simulink model "ideal_ballnbeam"  (R2020b)
settings: Solver=ode15s  StartTime=0.0  StopTime=100  RelTol=1e-3
undefined symbols (not defined in the file): ball, ballnbeam, const, mech
settings Model: Creator=Utente  LastModifiedBy=Utente

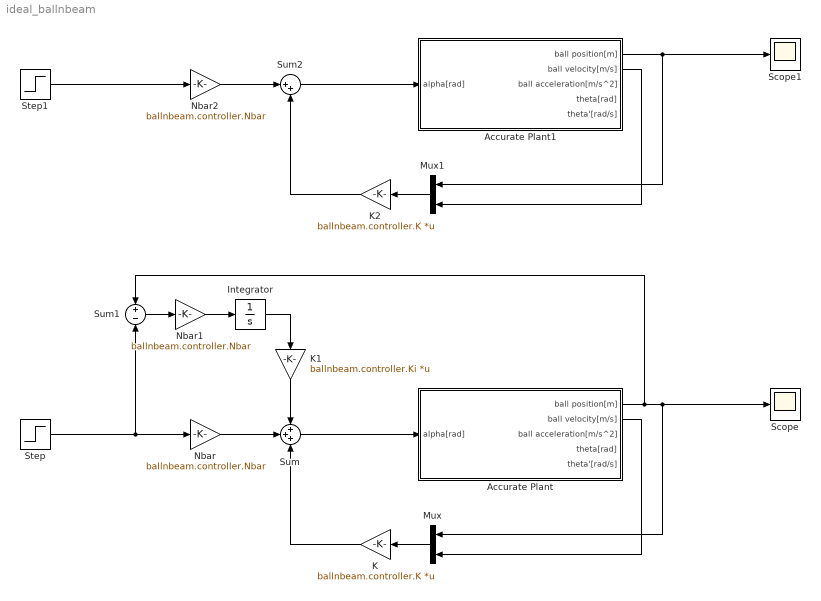
== system ideal_ballnbeam ==
  Accurate Plant : Subsystem
  Accurate Plant1 : Subsystem
  Integrator : Integrator
  K : Gain  Gain=ballnbeam.controller.K  Multiplication=Matrix(K*u)
  K1 : Gain  Gain=ballnbeam.controller.Ki  Multiplication=Matrix(K*u)
  K2 : Gain  Gain=ballnbeam.controller.K  Multiplication=Matrix(K*u)
  Mux : Mux  Inputs=2
  Mux1 : Mux  Inputs=2
  Nbar : Gain  Gain=ballnbeam.controller.Nbar
  Nbar1 : Gain  Gain=ballnbeam.controller.Nbar
  Nbar2 : Gain  Gain=ballnbeam.controller.Nbar
  Scope : Scope
  Scope1 : Scope
  Step : Step  Time=0  After=0.25  SampleTime=0
  Step1 : Step  Time=0  After=0.25  SampleTime=0
  Sum : Sum  Inputs=+++
  Sum1 : Sum  Inputs=+|-
  Sum2 : Sum  Inputs=|++
  wires:
  Accurate Plant/1(ball position[m]) -> Mux/1, Scope/1, Sum1/1
  Sum/1 -> Accurate Plant/1(alpha[rad])
  Mux/1 -> K/1
  Accurate Plant/2(ball velocity[m/s]) -> Mux/2
  Sum1/1 -> Nbar1/1
  Integrator/1 -> K1/1
  K/1 -> Sum/3
  Step/1 -> Nbar/1, Sum1/2
  K1/1 -> Sum/1
  Nbar1/1 -> Integrator/1
  Nbar/1 -> Sum/2
  Step1/1 -> Nbar2/1
  K2/1 -> Sum2/2
  Accurate Plant1/1(ball position[m]) -> Mux1/1, Scope1/1
  Accurate Plant1/2(ball velocity[m/s]) -> Mux1/2
  Sum2/1 -> Accurate Plant1/1(alpha[rad])
  Mux1/1 -> K2/1
  Nbar2/1 -> Sum2/1

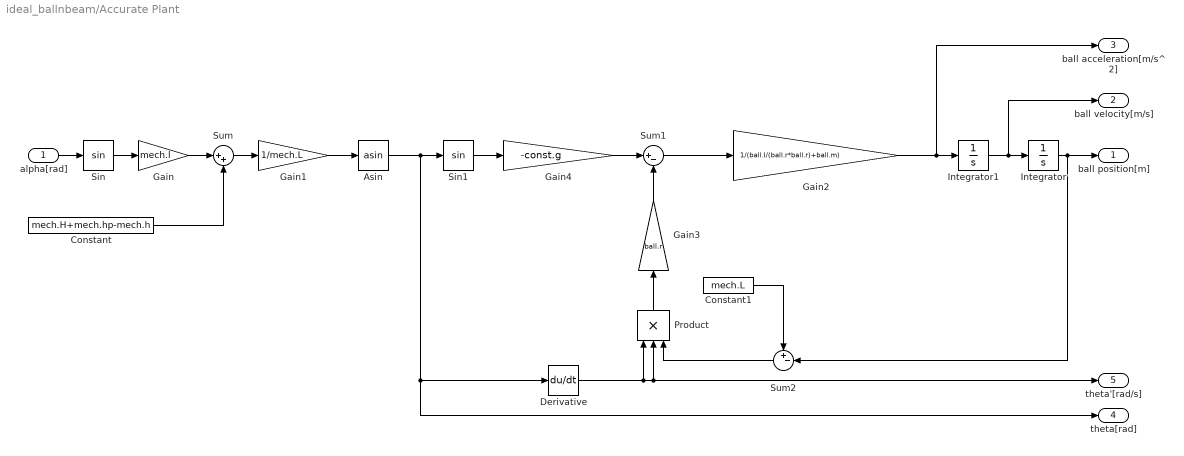
== system ideal_ballnbeam/Accurate Plant ==
  alpha[rad] : Inport
  Asin : Trigonometry  Operator=asin
  Constant : Constant  Value=mech.H+mech.hp-mech.h
  Constant1 : Constant  Value=mech.L
  Derivative : Derivative
  Gain : Gain  Gain=mech.l
  Gain1 : Gain  Gain=1/mech.L
  Gain2 : Gain  Gain=1/(ball.I/(ball.r*ball.r)+ball.m)
  Gain3 : Gain  Gain=ball.r
  Gain4 : Gain  Gain=-const.g
  Integrator : Integrator
  Integrator1 : Integrator
  Product : Product  Inputs=3
  Sin : Trigonometry
  Sin1 : Trigonometry
  Sum : Sum  Inputs=|++
  Sum1 : Sum  Inputs=|+-
  Sum2 : Sum  Inputs=+-|
  ball position[m] : Outport
  ball velocity[m/s] : Outport  Port=2
  ball acceleration[m/s^2] : Outport  Port=3
  theta[rad] : Outport  Port=4
  theta'[rad/s] : Outport  Port=5
  wires:
  Integrator/1 -> Sum2/2, ball position[m]/1
  Integrator1/1 -> ball velocity[m/s]/1, Integrator/1
  Gain2/1 -> ball acceleration[m/s^2]/1, Integrator1/1
  Gain1/1 -> Asin/1
  Gain/1 -> Sum/1
  Sum/1 -> Gain1/1
  alpha[rad]/1 -> Sin/1
  Constant/1 -> Sum/2
  Sin/1 -> Gain/1
  Asin/1 -> Derivative/1, theta[rad]/1, Sin1/1
  Derivative/1 -> Product/1, theta'[rad/s]/1, Product/2
  Product/1 -> Gain3/1
  Gain3/1 -> Sum1/2
  Sum1/1 -> Gain2/1
  Sin1/1 -> Gain4/1
  Gain4/1 -> Sum1/1
  Sum2/1 -> Product/3
  Constant1/1 -> Sum2/1

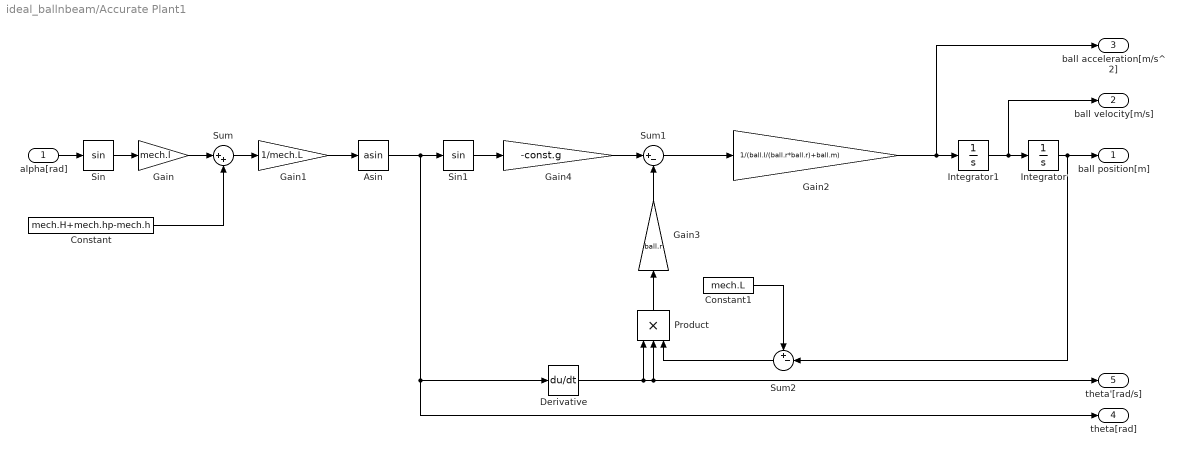
== system ideal_ballnbeam/Accurate Plant1 ==
  alpha[rad] : Inport
  Asin : Trigonometry  Operator=asin
  Constant : Constant  Value=mech.H+mech.hp-mech.h
  Constant1 : Constant  Value=mech.L
  Derivative : Derivative
  Gain : Gain  Gain=mech.l
  Gain1 : Gain  Gain=1/mech.L
  Gain2 : Gain  Gain=1/(ball.I/(ball.r*ball.r)+ball.m)
  Gain3 : Gain  Gain=ball.r
  Gain4 : Gain  Gain=-const.g
  Integrator : Integrator
  Integrator1 : Integrator
  Product : Product  Inputs=3
  Sin : Trigonometry
  Sin1 : Trigonometry
  Sum : Sum  Inputs=|++
  Sum1 : Sum  Inputs=|+-
  Sum2 : Sum  Inputs=+-|
  ball position[m] : Outport
  ball velocity[m/s] : Outport  Port=2
  ball acceleration[m/s^2] : Outport  Port=3
  theta[rad] : Outport  Port=4
  theta'[rad/s] : Outport  Port=5
  wires:
  Integrator/1 -> Sum2/2, ball position[m]/1
  Integrator1/1 -> ball velocity[m/s]/1, Integrator/1
  Gain2/1 -> ball acceleration[m/s^2]/1, Integrator1/1
  Gain1/1 -> Asin/1
  Gain/1 -> Sum/1
  Sum/1 -> Gain1/1
  alpha[rad]/1 -> Sin/1
  Constant/1 -> Sum/2
  Sin/1 -> Gain/1
  Asin/1 -> Derivative/1, theta[rad]/1, Sin1/1
  Derivative/1 -> Product/1, theta'[rad/s]/1, Product/2
  Product/1 -> Gain3/1
  Gain3/1 -> Sum1/2
  Sum1/1 -> Gain2/1
  Sin1/1 -> Gain4/1
  Gain4/1 -> Sum1/1
  Sum2/1 -> Product/3
  Constant1/1 -> Sum2/1
